simulink model "local_sequencer"  (R2018b)
settings: Solver=FixedStepAuto  StartTime=0.0  StopTime=70  RelTol=1e-3
values from neighbouring files (symbols this model uses):
  eof = int32(2147483647)    [setup.m]
libraries: simulink x5, hdlsllib x4
settings Model: Creator=hiterd  LastModifiedBy=jayakumarav
settings DebuggingCC: LibraryContextMissingDiagnostic=none
settings SFSimCC: SimUseLocalCustomCode=off
settings RTWCC: RTWUseLocalCustomCode=off
settings ConfigComp: DVTestSuiteOptimization=CombinedObjectives (Nonlinear Extended)  DVSaveExpectedOutput=on

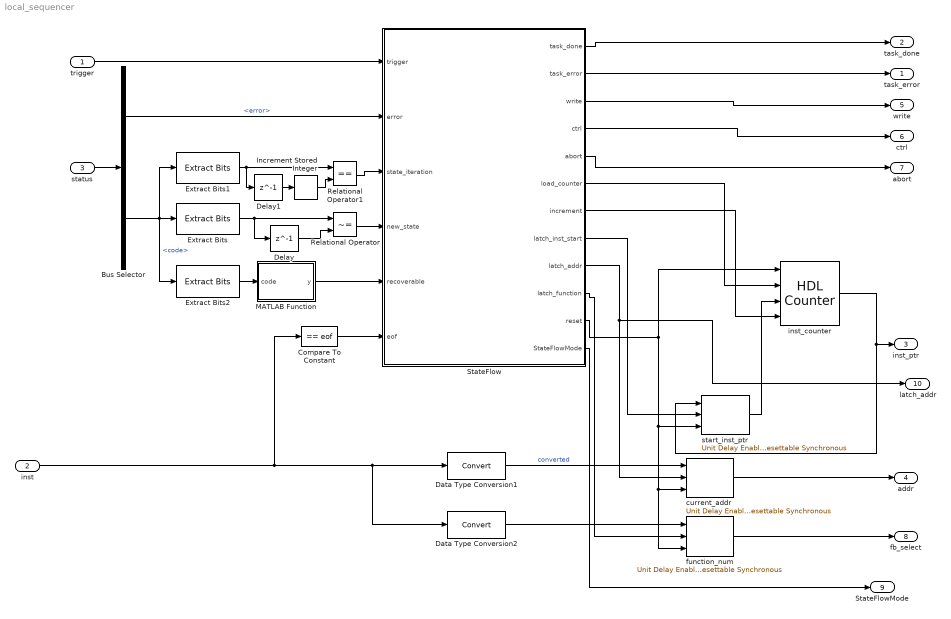
== system local_sequencer ==
  trigger : Inport  OutDataTypeStr=boolean  SampleTime=1
  inst : Inport  Port=2  OutDataTypeStr=task_inst_data_type  SampleTime=1
  status : Inport  Port=3  OutDataTypeStr=Bus: fb_status  SampleTime=1
  Bus Selector : BusSelector  OutputSignals=error,code
  Compare To Constant : simulink/Logic and Bit Operations/Compare To Constant  relop===  const=eof  OutDataTypeStr=boolean
  Data Type Conversion1 : DataTypeConversion
  Data Type Conversion2 : DataTypeConversion
  Delay : Delay  DelayLength=1
  Delay1 : Delay  DelayLength=1
  Extract Bits : simulink/Logic and Bit Operations/Extract Bits  bitsToExtract=Range starting with most significant bit  numBits=4  bitIdxRange=[0 7]  outScalingMode=Treat bit field as an integer
      settings: SourceProductName=Simulink
  Extract Bits1 : simulink/Logic and Bit Operations/Extract Bits  bitsToExtract=Range of bits  numBits=4  bitIdxRange=[22 27]  outScalingMode=Treat bit field as an integer
      settings: SourceProductName=Simulink
  Extract Bits2 : simulink/Logic and Bit Operations/Extract Bits  bitsToExtract=Range ending with least significant bit  numBits=22  bitIdxRange=[22 27]  outScalingMode=Treat bit field as an integer
      settings: SourceProductName=Simulink
  Increment Stored Integer : simulink/Additional Math & Discrete/Additional Math: Increment - Decrement/Increment Stored Integer
      settings: SourceProductName=Simulink
  MATLAB Function : MATLAB Function  TreatAsAtomicUnit=on
  Relational Operator : RelationalOperator  Operator=~=  OutDataTypeStr=boolean  RndMeth=Nearest
  Relational Operator1 : RelationalOperator  Operator===  OutDataTypeStr=boolean  RndMeth=Nearest
  StateFlow : Stateflow chart  TreatAsAtomicUnit=on
  current_addr : hdlsllib/Discrete/Unit Delay Enabled Resettable Synchronous  InitialCondition=0  SampleTime=-1
      settings: SourceProductName=HDL Coder  SourceProductBaseCode=HD
  function_num : hdlsllib/Discrete/Unit Delay Enabled Resettable Synchronous  InitialCondition=0  SampleTime=-1
      settings: SourceProductName=HDL Coder  SourceProductBaseCode=HD
  inst_counter : hdlsllib/Sources/HDL Counter  CountType=Free running  CountInit=0  CountStep=1  CountMax=25  CountFromType=Initial value  CountFrom=0  CountResetPort=on  CountLoadPort=on  CountEnbPort=on  CountDirPort=off  CountDataType=Unsigned  CountWordLen=32  CountFracLen=0  CountSampTime=1
      settings: SourceProductBaseCode=HD
  start_inst_ptr : hdlsllib/Discrete/Unit Delay Enabled Resettable Synchronous  InitialCondition=0  SampleTime=-1
      settings: SourceProductName=HDL Coder  SourceProductBaseCode=HD
  task_error : Outport  OutDataTypeStr=boolean
  task_done : Outport  Port=2  OutDataTypeStr=boolean
  inst_ptr : Outport  Port=3  OutDataTypeStr=task_inst_ptr_type
  addr : Outport  Port=4  OutMin=[0]  OutDataTypeStr=task_memory_addr_type
  write : Outport  Port=5  OutDataTypeStr=boolean
  ctrl : Outport  Port=6  OutDataTypeStr=boolean
  abort : Outport  Port=7  OutDataTypeStr=boolean
  fb_select : Outport  Port=8  OutDataTypeStr=fb_select_type
  StateFlowMode : Outport  Port=9
  latch_addr : Outport  Port=10  OutMin=[0]  OutDataTypeStr=boolean
  wires:
  trigger/1 -> StateFlow/1(trigger)
  StateFlow/3(write) -> write/1
  StateFlow/1(task_done) -> task_done/1
  StateFlow/9(latch_addr) -> latch_addr/1, current_addr/2
  current_addr/1 -> addr/1
  StateFlow/10(latch_function) -> function_num/2
  inst_counter/1 -> start_inst_ptr/1, inst_ptr/1
  StateFlow/7(increment) -> inst_counter/4
  start_inst_ptr/1 -> inst_counter/3
  inst/1 -> Data Type Conversion1/1, Data Type Conversion2/1, Compare To Constant/1
  StateFlow/11(reset) -> function_num/3, current_addr/3, start_inst_ptr/3, inst_counter/1
  function_num/1 -> fb_select/1
  StateFlow/8(latch_inst_start) -> start_inst_ptr/2
  status/1 -> Bus Selector/1
  StateFlow/4(ctrl) -> ctrl/1
  Delay/1 -> Relational Operator/2
  Relational Operator/1 -> StateFlow/4(new_state)
  Bus Selector/2 -> Extract Bits2/1, Extract Bits1/1, Extract Bits/1  "<code>"
  Bus Selector/1 -> StateFlow/2(error)  "<error>"
  MATLAB Function/1(y) -> StateFlow/5(recoverable)
  StateFlow/5(abort) -> abort/1
  StateFlow/2(task_error) -> task_error/1
  Compare To Constant/1 -> StateFlow/6(eof)
  Extract Bits1/1 -> Delay1/1, Relational Operator1/1
  Delay1/1 -> Increment Stored Integer/1
  Increment Stored Integer/1 -> Relational Operator1/2
  Relational Operator1/1 -> StateFlow/3(state_iteration)
  Extract Bits2/1 -> MATLAB Function/1(code)
  Data Type Conversion2/1 -> function_num/1
  Data Type Conversion1/1 -> current_addr/1  "converted"
  StateFlow/12(StateFlowMode) -> StateFlowMode/1
  StateFlow/6(load_counter) -> inst_counter/2
  Extract Bits/1 -> Relational Operator/1, Delay/1

== stateflow chart local_sequencer/StateFlow ==
  settings: stateMachineType=MOORE_MACHINE  initializeOutput=1
  note: Make trigger and enable to chart?
  state INIT
    task_done = false;
    task_error = false;
    write = false;
    load_counter = false;
    ctrl = false;
    abort = false;
    increment = false;
    latch_inst_start = false;
    latch_addr = false;
    latch_function = false;
    reset = true;
  state FB_SELECT
    state LOAD_INST_START
      task_done = false;
      task_error = false;
      write = false;
      ctrl = false;
      abort = false;
      load_counter = true;
      increment = false;
      latch_inst_start = false;
      latch_addr = false;
      latch_function = false;
      reset = false;
    state LATCH_INST_START
      task_done = false;
      task_error = false;
      write = false;
      ctrl = false;
      abort = false;
      load_counter = false;
      increment = false;
      latch_inst_start = true;
      latch_addr = false;
      latch_function = true;
      reset = false;
    state INCREMENT_INST
      task_done = false;
      task_error = false;
      write = false;
      ctrl = false;
      abort = false;
      load_counter = false;
      increment = true;
      latch_inst_start = false;
      latch_addr = false;
      latch_function = false;
      reset = false;
    state INST_WAIT
      task_done = false;
      task_error = false;
      write = false;
      ctrl = false;
      abort = false;
      load_counter = false;
      increment = false;
      latch_inst_start = false;
      latch_addr = false;
      latch_function = false;
      reset = false;
    (default) -> LOAD_INST_START [order 1] : [recoverable]
    (default) -> LATCH_INST_START [order 2]
    LATCH_INST_START -> (junction 371)
    LOAD_INST_START -> (junction 371)
    (junction 371) -> FB_SELECT.INCREMENT_INST
    FB_SELECT.INCREMENT_INST -> FB_SELECT.INST_WAIT
  state FETCH
    state CTRL_LO
      task_done = false;
      task_error = false;
      write = false;
      ctrl = false;
      abort = false;
      load_counter = false;
      increment = false;
      latch_inst_start = false;
      latch_addr = false;
      latch_function = false;
      reset = false;
    state INCREMENT_INST
      task_done = false;
      task_error = false;
      write = false;
      ctrl = false;
      abort = false;
      load_counter = false;
      increment = true;
      latch_inst_start = false;
      latch_addr = false;
      latch_function = false;
      reset = false;
    state CTRL_HI
      task_done = false;
      task_error = false;
      write = false;
      ctrl = true;
      abort = false;
      load_counter = false;
      increment = false;
      latch_inst_start = false;
      latch_addr = false;
      latch_function = false;
      reset = false;
    state INST_WAIT
      task_done = false;
      task_error = false;
      write = false;
      ctrl = false;
      abort = false;
      load_counter = false;
      increment = false;
      latch_inst_start = false;
      latch_addr = false;
      latch_function = false;
      reset = false;
    state LATCH_ADDR
      task_done = false;
      task_error = false;
      write = false;
      ctrl = false;
      abort = false;
      load_counter = false;
      increment = false;
      latch_inst_start = false;
      latch_addr = true;
      latch_function = false;
      reset = false;
    state MEM_WAIT
      task_done = false;
      task_error = false;
      write = false;
      ctrl = false;
      abort = false;
      load_counter = false;
      increment = false;
      latch_inst_start = false;
      latch_addr = false;
      latch_function = false;
      reset = false;
    (default) -> FETCH.LATCH_ADDR
    FETCH.CTRL_LO -> FETCH.INCREMENT_INST
    FETCH.CTRL_HI -> FETCH.CTRL_LO
    FETCH.LATCH_ADDR -> MEM_WAIT
    MEM_WAIT -> FETCH.CTRL_HI
    FETCH.INCREMENT_INST -> FETCH.INST_WAIT
  state FB_EXECUTE
    state CTRL_HI
      task_done = false;
      task_error = false;
      write = false;
      ctrl = true;
      abort = false;
      load_counter = false;
      increment = false;
      latch_inst_start = false;
      latch_addr = false;
      latch_function = false;
      reset = false;
    state CTRL_LO
      task_done = false;
      task_error = false;
      write = false;
      ctrl = false;
      abort = false;
      load_counter = false;
      increment = false;
      latch_inst_start = false;
      latch_addr = false;
      latch_function = false;
      reset = false;
    (default) -> FB_EXECUTE.CTRL_HI
    FB_EXECUTE.CTRL_HI -> FB_EXECUTE.CTRL_LO
  state ERROR
    state CTRL_HI
      %set control and clear init
      task_done = false;
      task_error = false;
      write = false;
      ctrl = true;
      abort = false;
      load_counter = false;
      increment = false;
      latch_inst_start = false;
      latch_addr = false;
      latch_function = false;
      reset = false;
    state ABORT_CTRL_LO
      %task_error and init
      %unchanged
      task_done = false;
      task_error = task_error;
      write = false;
      ctrl = false;
      abort = false;
      load_counter = false;
      increment = false;
      latch_inst_start = false;
      latch_addr = false;
      latch_function = false;
      reset = false;
    state ABORT_CTRL_HI
      %set control, abort, and init
      task_done = false;
      task_error = true;
      write = false;
      ctrl = true;
      abort = true;
      load_counter = false;
      increment = false;
      latch_inst_start = false;
      latch_addr = false;
      latch_function = false;
      reset = false;
    (default) -> ERROR.CTRL_HI [order 1] : [recoverable]
    ERROR.CTRL_HI -> (junction 308)
    (default) -> ABORT_CTRL_HI [order 2]
    (junction 308) -> ABORT_CTRL_LO
    ABORT_CTRL_HI -> (junction 308)
  state WRITE
    state WRITE
      task_done = false;
      task_error = false;
      write = true;
      ctrl = false;
      abort = false;
      load_counter = false;
      increment = false;
      latch_inst_start = false;
      latch_addr = false;
      latch_function = false;
      reset = false;
    state INCREMENT_INST
      task_done = false;
      task_error = false;
      write = false;
      ctrl = false;
      abort = false;
      load_counter = false;
      increment = true;
      latch_inst_start = false;
      latch_addr = false;
      latch_function = false;
      reset = false;
    state CTRL_LO
      task_done = false;
      task_error = false;
      write = false;
      ctrl = false;
      abort = false;
      load_counter = false;
      increment = false;
      latch_inst_start = false;
      latch_addr = false;
      latch_function = false;
      reset = false;
    state CTRL_HI
      task_done = false;
      task_error = false;
      write = false;
      ctrl = true;
      abort = false;
      load_counter = false;
      increment = false;
      latch_inst_start = false;
      latch_addr = false;
      latch_function = false;
      reset = false;
    state LATCH_ADDR
      %latch current address
      task_done = false;
      task_error = false;
      write = false;
      ctrl = false;
      abort = false;
      load_counter = false;
      increment = false;
      latch_inst_start = false;
      latch_addr = true;
      latch_function = false;
      reset = false;
    state INST_WAIT
      task_done = false;
      task_error = false;
      write = false;
      ctrl = false;
      abort = false;
      load_counter = false;
      increment = false;
      latch_inst_start = false;
      latch_addr = false;
      latch_function = false;
      reset = false;
    (default) -> WRITE.LATCH_ADDR
    WRITE.LATCH_ADDR -> WRITE.CTRL_HI
    WRITE.CTRL_HI -> WRITE.CTRL_LO
    WRITE.WRITE -> WRITE.INCREMENT_INST
    WRITE.CTRL_LO -> WRITE.WRITE
    WRITE.INCREMENT_INST -> WRITE.INST_WAIT
  state FB_DONE
    state CTRL_HI
      task_done = false;
      task_error = false;
      write = false;
      ctrl = true;
      abort = false;
      load_counter = false;
      increment = false;
      latch_inst_start = false;
      latch_addr = false;
      latch_function = false;
      reset = false;
    state CTRL_LO
      task_done = false;
      task_error = false;
      write = false;
      ctrl = false;
      abort = false;
      load_counter = false;
      increment = false;
      latch_inst_start = false;
      latch_addr = false;
      latch_function = false;
      reset = false;
    (default) -> FB_DONE.CTRL_HI
    FB_DONE.CTRL_HI -> FB_DONE.CTRL_LO
  state TASK_DONE
    %signal task done
    task_done = true;
    task_error = false;
    write = false;
    ctrl = false;
    abort = false;
    load_counter = false;
    increment = false;
    latch_inst_start = false;
    latch_addr = false;
    latch_function = false;
    reset = false;
  FB_SELECT.INST_WAIT -> FETCH
  WRITE.INST_WAIT -> (junction 207)
  FB_DONE.CTRL_LO -> (junction 315) : [new_state]
  FB_EXECUTE.CTRL_LO -> WRITE : [new_state]
  FETCH.INST_WAIT -> (junction 204)
  ABORT_CTRL_LO -> (junction 220)
  (default) -> INIT
  (junction 220) -> INIT [order 2] : [~trigger]
  TASK_DONE -> INIT : [~trigger]
  INIT -> FB_SELECT : [trigger]
  (junction 220) -> FB_SELECT [order 1] : [recoverable]
  (junction 315) -> FB_SELECT [order 2]
  FETCH -> (junction 197)
  (junction 204) -> FETCH [order 2] : [state_iteration]
  (junction 204) -> FB_EXECUTE [order 1] : [new_state]
  FB_EXECUTE -> (junction 197)
  (junction 197) -> ERROR : [error]
  WRITE -> (junction 197)
  (junction 207) -> WRITE [order 2] : [state_iteration]
  (junction 207) -> FB_DONE [order 1] : [new_state]
  (junction 315) -> TASK_DONE [order 1] : [eof]
  data: task_done output boolean; task_error output boolean; write output boolean; ctrl output boolean; abort output boolean; load_counter output boolean; increment output boolean; latch_inst_start output boolean; latch_addr output boolean; latch_function output boolean; trigger input boolean; error input boolean; state_iteration input boolean; reset output boolean; new_state input boolean; recoverable input boolean; eof input boolean; StateFlowMode output Enum: StateFlowModeType

== matlab function local_sequencer/MATLAB Function ==
  data: code input; y output
function y = recoverable(code)
%#codegen

if(code)
    y = true;
else
    y = false;
end
